simulink model "dynamics"  (R2023a)
settings: Solver=ode4  StartTime=0.0  StopTime=2*86400  FixedStep=dt  RelTol=1e-3
undefined symbols (not defined in the file): plant
settings Model: Creator=ndelurgio  LastModifiedBy=hugobuurmeijer

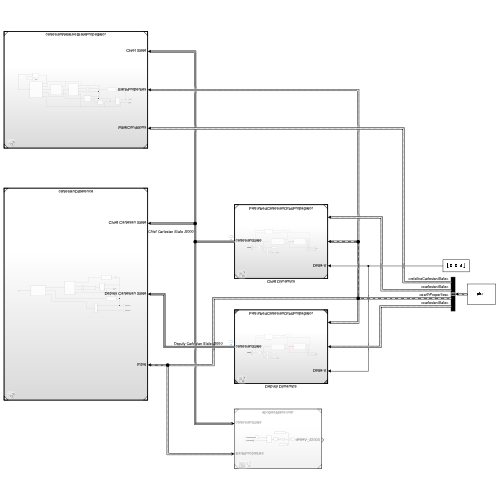
[thumbnail: Simulink's stored preview of the top-level diagram]
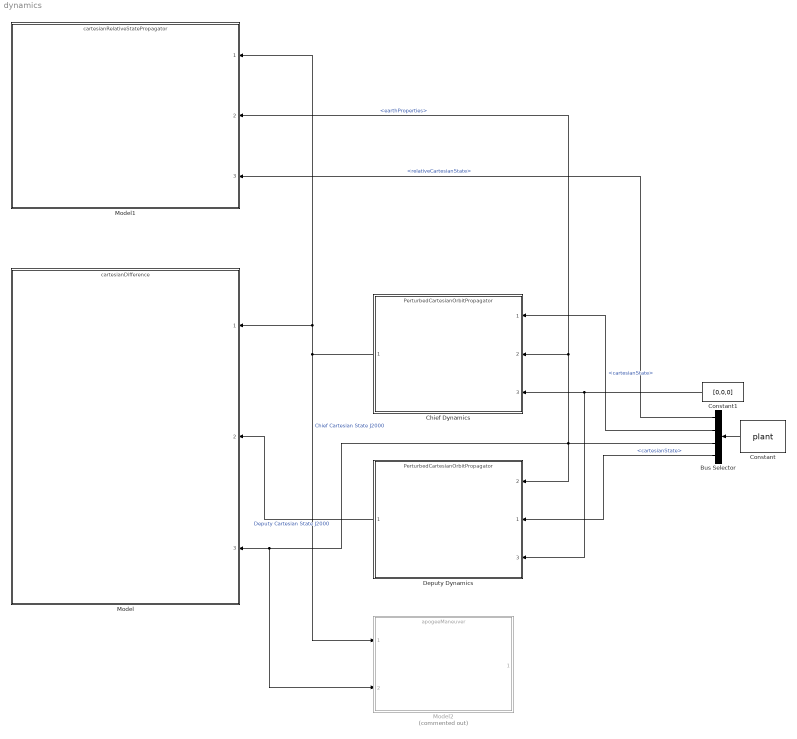
== system dynamics ==
  Bus Selector : BusSelector  OutputSignals=deputy.initialConditions.relativeCartesianState,chief.initialConditions.cartesianState,environment.earthProperties,deputy.initialConditions.cartesianState
  Chief Dynamics : ModelReference  ModelNameDialog=PerturbedCartesianOrbitPropagator.slx  SimulationMode=Normal  ModelReferenceVersion=1.44
  Constant : Constant  Value=plant  OutDataTypeStr=Bus: plantBus
  Constant1 : Constant  Value=[0,0,0]
  Deputy Dynamics : ModelReference  ModelNameDialog=PerturbedCartesianOrbitPropagator.slx  SimulationMode=Normal  ModelReferenceVersion=1.44
      settings: PortSchema="{\"entries\":[{\"content\":{\"sides\":[{\"content\":{\"connectorIds\":[\"In2\",\"In1\",\"In3\"]},\"type\":\"ConnectorPlacement.EquallySpacedRectSide\",\"uuid\":\"4c211678-740f-40f0-887b-605a3322d7cb\"},{\"content\":{\"connectorIds\":[\"Out1\"],\"side\":\"RIGHT\"},\"type\":\"ConnectorPlacement.EquallySpacedRectSide\",\"uuid\":\"7e8d6e44-a7a2-4633-9eac-45eb2a30ed1c\"},{\"content\":{\"side\":\"TOP\"},\"type\":\"ConnectorPlacement.EquallySpacedRectSide\",\"uuid\":\"00358f8f-509c-447f-b607-9e6e4b9aa7b5\"}]},\"type\":\"ConnectorPlacement.EquallySpacedConnector\",\"uuid\":\"f8258235-53bd-4241-8f5f-7f5c3c0a64eb\"}],\"packageUris\":[\"http://schema.mathworks.com/mf0/Connector/R2020b\"],\"version\":\"1.0\"}"
  Model : ModelReference  ModelNameDialog=cartesianDifference  SimulationMode=Normal  ModelReferenceVersion=1.27
  Model1 : ModelReference  ModelNameDialog=cartesianRelativeStatePropagator  SimulationMode=Normal  ModelReferenceVersion=1.34
  Model2 : ModelReference  Commented=on  ModelNameDialog=apogeeManeuver.slx  SimulationMode=Normal  ModelReferenceVersion=1.15
  wires:
  Constant/1 -> Bus Selector/1
  Bus Selector/3 -> Model2/2, Model/3, Chief Dynamics/2, Model1/2, Deputy Dynamics/2  "<earthProperties>"
  Bus Selector/2 -> Chief Dynamics/1  "<cartesianState>"
  Bus Selector/4 -> Deputy Dynamics/1  "<cartesianState>"
  Chief Dynamics/1 -> Model2/1, Model1/1, Model/1  "Chief Cartesian State J2000"
  Deputy Dynamics/1 -> Model/2  "Deputy Cartesian State J2000"
  Bus Selector/1 -> Model1/3  "<relativeCartesianState>"
  Constant1/1 -> Deputy Dynamics/3, Chief Dynamics/3
